simulink model "ManualCommandModule"  (R2020b)
settings: Solver=VariableStepAuto  StartTime=0.0  StopTime=10.0  RelTol=1e-3
model workspace (MAT data in the model file):
  cam_control_gain = 1
  l_stick_x_gain = 1
  l_stick_y_gain = 1
  r_stick_x_gain = 1
  r_stick_y_gain = 1
settings Model: Creator=macra  LastModifiedBy=macra

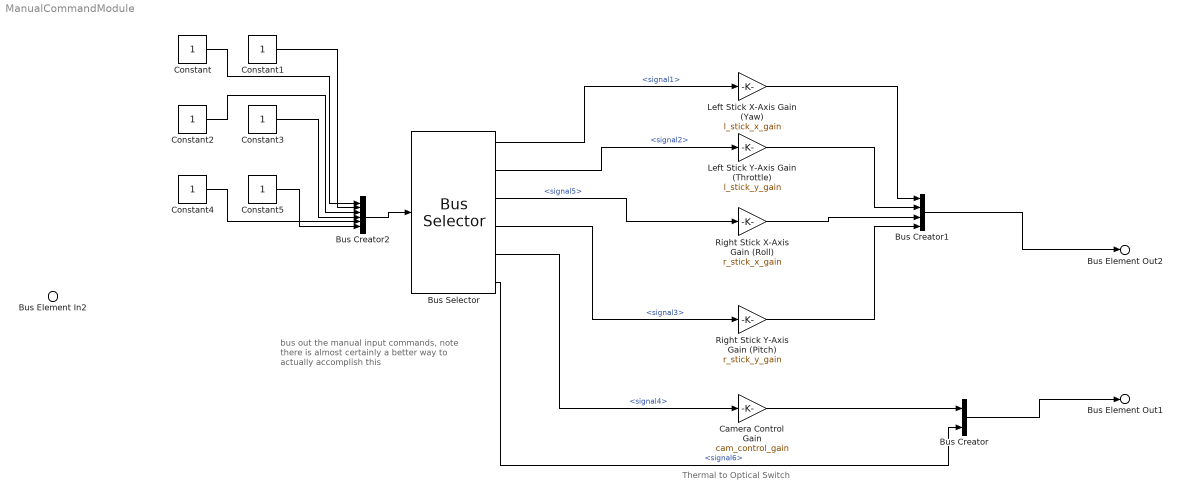
== system ManualCommandModule ==
  note: Thermal to Optical Switch
  note: bus out the manual input commands,
      | note there is almost certainly a better way
      | to actually accomplish this
  Bus Element In2 : Inport  PortName=Input Commands
  Bus Creator : BusCreator  Inputs=2
  Bus Creator1 : BusCreator  Inputs=4
  Bus Creator2 : BusCreator  Inputs=6
  Bus Selector : BusSelector  OutputSignals=signal1,signal2,signal5,signal3,signal4,signal6
  Camera Control Gain : Gain  Gain=cam_control_gain
  Constant{,1..5} (6 alike) : Constant
  Left Stick X-Axis Gain (Yaw) : Gain  Gain=l_stick_x_gain
  Left Stick Y-Axis Gain (Throttle) : Gain  Gain=l_stick_y_gain
  Right Stick X-Axis Gain (Roll) : Gain  Gain=r_stick_x_gain
  Right Stick Y-Axis Gain (Pitch) : Gain  Gain=r_stick_y_gain
  Bus Element Out2 : Outport  PortName=Throttle Control
  Bus Element Out1 : Outport  Port=2  PortName=Camera Control
  wires:
  Camera Control Gain/1 -> Bus Creator/1
  Bus Creator/1 -> Bus Element Out1/1
  Left Stick X-Axis Gain (Yaw)/1 -> Bus Creator1/1
  Right Stick Y-Axis Gain (Pitch)/1 -> Bus Creator1/4
  Left Stick Y-Axis Gain (Throttle)/1 -> Bus Creator1/2
  Right Stick X-Axis Gain (Roll)/1 -> Bus Creator1/3
  Bus Creator1/1 -> Bus Element Out2/1
  Bus Selector/1 -> Left Stick X-Axis Gain (Yaw)/1  "<signal1>"
  Bus Selector/2 -> Left Stick Y-Axis Gain (Throttle)/1  "<signal2>"
  Bus Selector/4 -> Right Stick Y-Axis Gain (Pitch)/1  "<signal3>"
  Bus Selector/5 -> Camera Control Gain/1  "<signal4>"
  Bus Selector/3 -> Right Stick X-Axis Gain (Roll)/1  "<signal5>"
  Bus Selector/6 -> Bus Creator/2  "<signal6>"
  Bus Creator2/1 -> Bus Selector/1
  Constant/1 -> Bus Creator2/1
  Constant1/1 -> Bus Creator2/2
  Constant2/1 -> Bus Creator2/3
  Constant3/1 -> Bus Creator2/4
  Constant4/1 -> Bus Creator2/5
  Constant5/1 -> Bus Creator2/6
